simulink model "AltitudeController"  (Simulink 8.5)
settings: Solver=ode45  StartTime=0.0  StopTime=10.0  RelTol=1e-3
settings Model: Creator=teme  LastModifiedBy=teme
settings DataIOCC: SignalLoggingSaveFormat=Dataset
settings OptimizationCC: ExpressionDepthLimit=128
settings DebuggingCC: UnderspecifiedInitializationDetection=Simplified  MergeDetectMultiDrivingBlocksExec=error  FcnCallInpInsideContextMsg=EnableAllAsError  StateNameClashWarn=none
settings GRTTargetCC: CombineOutputUpdateFcns=on  GRTInterface=off

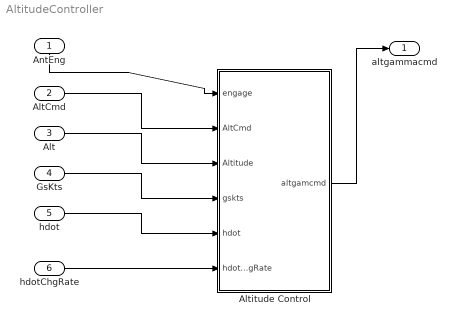
== system AltitudeController ==
  AntEng : Inport  OutDataTypeStr=boolean
  AltCmd : Inport  Port=2  OutDataTypeStr=double
  Alt : Inport  Port=3  OutDataTypeStr=double
  GsKts : Inport  Port=4  OutDataTypeStr=double
  hdot : Inport  Port=5  OutDataTypeStr=double
  hdotChgRate : Inport  Port=6  OutDataTypeStr=double
  Altitude Control : Subsystem  RequirementInfo={'other' '..\..\tcm_requirements.docx' '@Simulink_requirement_item_14' 'true' 'Altitude Control' '' } %GIDa_740ef422_46e2_47bc_9a8b_72c78cd9c99f
  altgammacmd : Outport
  wires:
  Alt/1 -> Altitude Control/3(Altitude)
  AltCmd/1 -> Altitude Control/2(AltCmd)
  Altitude Control/1(altgamcmd) -> altgammacmd/1
  hdot/1 -> Altitude Control/5(hdot)
  GsKts/1 -> Altitude Control/4(gskts)
  AntEng/1 -> Altitude Control/1(engage)
  hdotChgRate/1 -> Altitude Control/6(hdotChgRate)

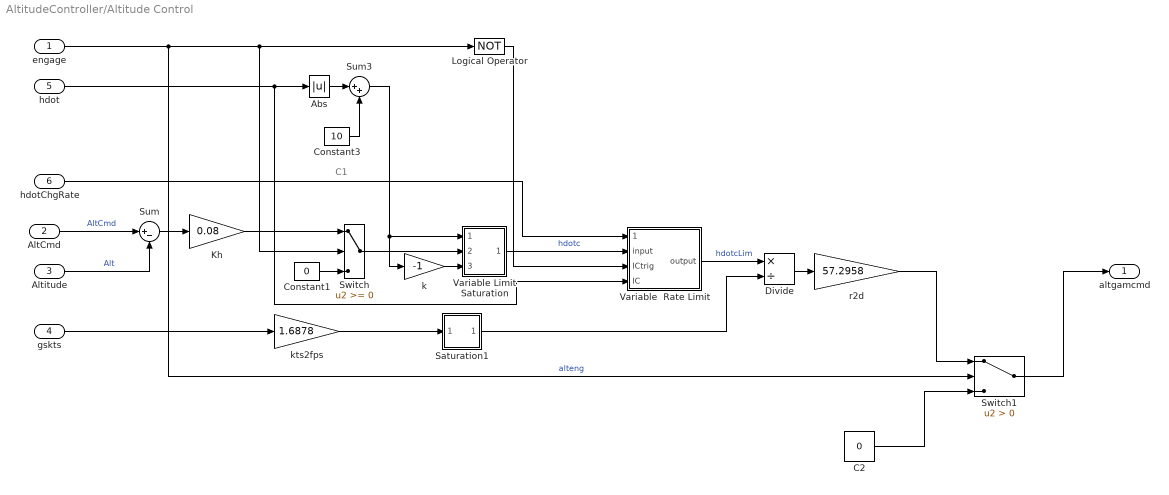
== system AltitudeController/Altitude Control ==
  note: C1
  engage : Inport  RequirementInfo={} %GIDa_557f6770_9a6e_476f_9a21_bb9d521836db
  AltCmd : Inport  RequirementInfo={} %GIDa_1e392055_7c94_4c29_8b89_db81cd353d5d  Port=2
  Altitude : Inport  RequirementInfo={} %GIDa_bf7346ae_e47b_4d44_a9c1_a0d50ca48ef2  Port=3
  gskts : Inport  RequirementInfo={} %GIDa_686454f6_496c_4fdc_b1cb_6fde9ae3adb0  Port=4
  hdot : Inport  RequirementInfo={} %GIDa_3f861779_66dc_4c47_9b90_18f5db182502  Port=5
  hdotChgRate : Inport  Port=6
  Abs : Abs  RequirementInfo={} %GIDa_d7399883_42b8_44b8_8349_c619770e0c25  SaturateOnIntegerOverflow=on
  C2 : Constant  Value=0
  Constant1 : Constant  RequirementInfo={} %GIDa_847c63d8_7344_4667_8a33_b64a5087f0ec  Value=0
  Constant3 : Constant  RequirementInfo={} %GIDa_52899424_6ad7_47eb_bcc3_39bfc1eb81dd  Value=10
  Divide : Product  RequirementInfo={} %GIDa_4bef3e62_b463_4fea_8d10_5624b4059a70  Inputs=*/
  Kh : Gain  RequirementInfo={} %GIDa_ec8c100e_af76_4bb9_91d7_1fe1755bb897  Gain=0.08
  Logical Operator : Logic  RequirementInfo={} %GIDa_18f4fb3f_cd6d_4c97_9f9d_4640039c7a25  Operator=NOT
  Saturation1 : Subsystem  RequirementInfo={} %GIDa_b2518338_6b94_4909_accf_11943b3fa4df  TreatAsAtomicUnit=on
  Sum : Sum  RequirementInfo={} %GIDa_503e18fd_82fb_4f2c_904f_c7f2be08a3a9  Inputs=|+-
  Sum3 : Sum  RequirementInfo={} %GIDa_dd07c7d5_8f14_4e2d_abb7_7b4d38d491f7  Inputs=|++  SaturateOnIntegerOverflow=on  InputSameDT=on  OutDataTypeStr=Inherit: Same as first input
  Switch : Switch  RequirementInfo={} %GIDa_af9c748a_ed48_4391_a443_9819472c09a0
  Switch1 : Switch  Criteria=u2 > Threshold
  Variable  Rate Limit : Subsystem  RequirementInfo={} %GIDa_5c0e3f11_92e5_41c1_8608_c204ac5cdc78  TreatAsAtomicUnit=on
  Variable Limit Saturation : Subsystem  RequirementInfo={} %GIDa_669ab400_27d0_4585_935c_23de659fc0f3  TreatAsAtomicUnit=on
  k : Gain  RequirementInfo={} %GIDa_be88b67b_02f7_4591_968f_d8b4e507b571  Gain=-1
  kts2fps : Gain  RequirementInfo={} %GIDa_e8e6cf54_89a4_40bf_8597_30ca384472f5  Gain=1.6878
  r2d : Gain  RequirementInfo={} %GIDa_359d04be_a8d5_48b7_9da9_7238e8e77903  Gain=57.2958
  altgamcmd : Outport  RequirementInfo={} %GIDa_e2872f4d_8dba_49af_8e9f_1e25a3d3f6dd
  wires:
  Sum/1 -> Kh/1
  AltCmd/1 -> Sum/1  "AltCmd"
  Altitude/1 -> Sum/2  "Alt"
  hdot/1 -> Variable  Rate Limit/4(IC), Abs/1
  Abs/1 -> Sum3/1
  Constant3/1 -> Sum3/2
  k/1 -> Variable Limit Saturation/3(Lo_lim)
  Sum3/1 -> k/1, Variable Limit Saturation/1(up_lim)
  engage/1 -> Switch1/2, Switch/2, Logical Operator/1  "alteng"
  gskts/1 -> kts2fps/1
  Divide/1 -> r2d/1
  r2d/1 -> Switch1/1
  Logical Operator/1 -> Variable  Rate Limit/3(ICtrig)
  Variable Limit Saturation/1(Out1) -> Variable  Rate Limit/2(input)  "hdotc"
  hdotChgRate/1 -> Variable  Rate Limit/1(ratelim)
  Variable  Rate Limit/1(output) -> Divide/1  "hdotcLim"
  kts2fps/1 -> Saturation1/1(SigIn)
  Saturation1/1(Out1) -> Divide/2
  Switch/1 -> Variable Limit Saturation/2(SigIn)
  Kh/1 -> Switch/1
  Constant1/1 -> Switch/3
  Switch1/1 -> altgamcmd/1
  C2/1 -> Switch1/3

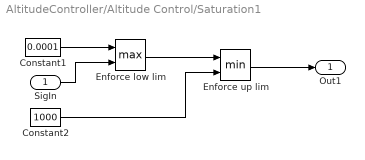
== system AltitudeController/Altitude Control/Saturation1 ==
  SigIn : Inport  RequirementInfo={} %GIDa_2aa6b3a0_984e_46ef_bb87_8deb7441b884
  Constant1 : Constant  RequirementInfo={} %GIDa_fedebcfc_196b_4714_887b_1f4ed602e269  Value=0.0001
  Constant2 : Constant  RequirementInfo={} %GIDa_416eef41_e100_4fef_93f4_04c4f859f011  Value=1000
  Enforce low lim : MinMax  RequirementInfo={} %GIDa_92c2e612_ea38_4c87_90b6_b001e0a05d74  Function=max  Inputs=2
  Enforce up lim : MinMax  RequirementInfo={} %GIDa_cc71b9aa_38c8_493a_922b_7237233e29a8  Inputs=2
  Out1 : Outport  RequirementInfo={} %GIDa_acd9a893_5404_43ad_a31c_e335c8441e29
  wires:
  Constant1/1 -> Enforce low lim/1
  SigIn/1 -> Enforce low lim/2
  Enforce low lim/1 -> Enforce up lim/1
  Constant2/1 -> Enforce up lim/2
  Enforce up lim/1 -> Out1/1

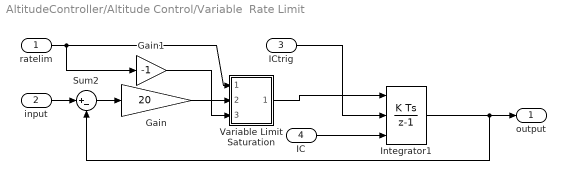
== system AltitudeController/Altitude Control/Variable  Rate Limit ==
  ratelim : Inport  RequirementInfo={} %GIDa_cebf8206_0991_4601_a693_e203a032dd60
  input : Inport  RequirementInfo={} %GIDa_1c42cf35_0a2c_4f00_a563_a653f4d148bc  Port=2  OutDataTypeStr=double
  ICtrig : Inport  RequirementInfo={} %GIDa_3275acdd_f2c7_434b_9677_e3cbf374fb67  Port=3
  IC : Inport  RequirementInfo={} %GIDa_0cbf00f5_4997_486f_9010_80b0a0243597  Port=4
  Gain : Gain  RequirementInfo={} %GIDa_eb981680_0415_4cd9_a42f_e63c1cec1621  Gain=20  SaturateOnIntegerOverflow=on  OutDataTypeStr=Inherit: Same as input  ParamDataTypeStr=Inherit: Same as input
  Gain1 : Gain  RequirementInfo={} %GIDa_a00c9a93_c1be_4be6_b4e3_8479bb90fd91  Gain=-1  SaturateOnIntegerOverflow=on  OutDataTypeStr=Inherit: Same as input  ParamDataTypeStr=Inherit: Same as input
  Integrator1 : DiscreteIntegrator  ExternalReset=level  InitialConditionSource=external  SampleTime=0.1  mask(DiscretizedDiscreteIntegrator){}
      mask init:
      | %zoh
  Sum2 : Sum  RequirementInfo={} %GIDa_882c640c_3bb5_4d7f_9311_9058c90f15b2  Inputs=|+-  SaturateOnIntegerOverflow=on
  Variable Limit Saturation : Subsystem  RequirementInfo={} %GIDa_1d312144_7e75_4364_a062_ba2ab73ad68e  TreatAsAtomicUnit=on
  output : Outport  RequirementInfo={} %GIDa_fe7b047d_58d9_46fc_8b53_9297abd7814c
  wires:
  Sum2/1 -> Gain/1
  Gain/1 -> Variable Limit Saturation/2(SigIn)
  ratelim/1 -> Gain1/1, Variable Limit Saturation/1(up_lim)
  Gain1/1 -> Variable Limit Saturation/3(Lo_lim)
  Integrator1/1 -> Sum2/2, output/1
  input/1 -> Sum2/1
  ICtrig/1 -> Integrator1/2
  IC/1 -> Integrator1/3
  Variable Limit Saturation/1(Out1) -> Integrator1/1

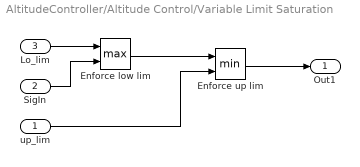
== system AltitudeController/Altitude Control/Variable Limit Saturation ==
  up_lim : Inport  RequirementInfo={} %GIDa_d20f7e48_25ba_49cb_bf86_675adf8748db
  SigIn : Inport  RequirementInfo={} %GIDa_761018a0_09ef_4028_9b40_731fe96a27cf  Port=2
  Lo_lim : Inport  RequirementInfo={} %GIDa_b6987e71_88fd_49d9_85dd_b44347a16467  Port=3
  Enforce low lim : MinMax  RequirementInfo={} %GIDa_ddd24ed5_9bb9_46fd_9043_f11ab698045a  Function=max  Inputs=2
  Enforce up lim : MinMax  RequirementInfo={} %GIDa_9e00fa09_18fb_4599_be11_f0c27ff3e824  Inputs=2
  Out1 : Outport  RequirementInfo={} %GIDa_7e9e4c58_88ea_4921_a313_52949ff005ba
  wires:
  Lo_lim/1 -> Enforce low lim/1
  SigIn/1 -> Enforce low lim/2
  Enforce low lim/1 -> Enforce up lim/1
  up_lim/1 -> Enforce up lim/2
  Enforce up lim/1 -> Out1/1

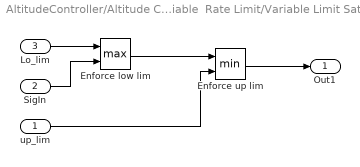
== system AltitudeController/Altitude Control/Variable  Rate Limit/Variable Limit Saturation ==
  up_lim : Inport  RequirementInfo={} %GIDa_70f2291e_942c_4be6_b3e0_e702a6f70818
  SigIn : Inport  RequirementInfo={} %GIDa_d51bfb00_2972_469b_897b_dcfde5f6a677  Port=2
  Lo_lim : Inport  RequirementInfo={} %GIDa_74e7c2ee_bf57_4296_b0b9_ff0672f27d70  Port=3
  Enforce low lim : MinMax  RequirementInfo={} %GIDa_73517a37_56ce_464d_8480_b6eda856e425  Function=max  Inputs=2
  Enforce up lim : MinMax  RequirementInfo={} %GIDa_2fa4640f_4bac_4541_b723_0ca232902dbb  Inputs=2
  Out1 : Outport  RequirementInfo={} %GIDa_85021c4c_80d3_49b2_aa67_6da309562141
  wires:
  Enforce up lim/1 -> Out1/1
  up_lim/1 -> Enforce up lim/2
  Enforce low lim/1 -> Enforce up lim/1
  SigIn/1 -> Enforce low lim/2
  Lo_lim/1 -> Enforce low lim/1
